simulink subsystem "actuator"  (R2024b)
settings: Solver=VariableStepAuto  StartTime=0.0  StopTime=10.0  RelTol=1e-3
undefined symbols (not defined in the file or in its folder): SERVO_TC
settings Model: Creator=yevge  LastModifiedBy=Aiden Gaydos

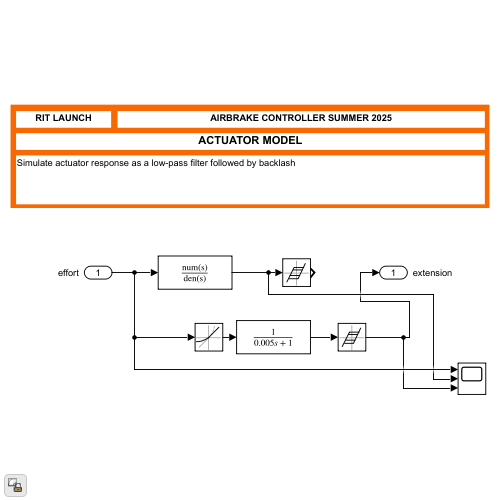
[thumbnail: Simulink's stored preview of the top-level diagram]
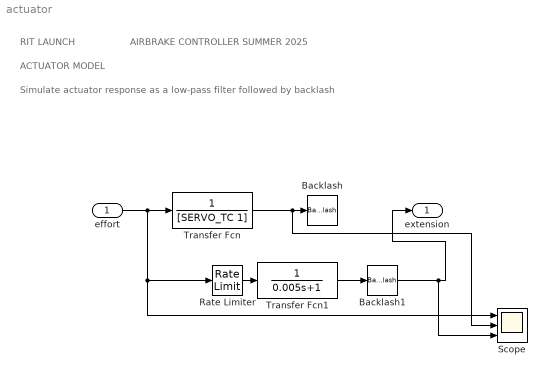
== system actuator ==
  note: RIT LAUNCH
  note: ACTUATOR MODEL
  note: Simulate actuator response as a low-pass filter followed by backlash
  note: AIRBRAKE CONTROLLER SUMMER 2025
  effort : Inport
  Backlash : Backlash  BacklashWidth=SERVO_BL
  Backlash1 : Backlash  BacklashWidth=SERVO_BL
  Rate Limiter : RateLimiter  RisingSlewLimit=6.25  FallingSlewLimit=-6.25
  Scope : Scope  NumInputPorts=3
  Transfer Fcn : TransferFcn  Denominator=[SERVO_TC 1]  ContinuousStateAttributes='actuator'
  Transfer Fcn1 : TransferFcn  Denominator=[0.005 1]  ContinuousStateAttributes='actuator'
  extension : Outport
  wires:
  Transfer Fcn/1 -> Backlash/1, Scope/2
  Rate Limiter/1 -> Transfer Fcn1/1
  Backlash1/1 -> extension/1, Scope/3
  Transfer Fcn1/1 -> Backlash1/1
  effort/1 -> Transfer Fcn/1, Scope/1, Rate Limiter/1
